simulink library "VIS_LIB"  (Simulink 8.6)
settings: Solver=ode45  StartTime=0.0  StopTime=10.0  RelTol=1e-3
undefined symbols (not defined in the file): AC, SIXOSEM_F_WD_AC_MASTER
libraries: cdsFilt x376, cdsEpicsOut x253, cdsEpicsIn x179, cdsTP x123, VIS_LIB x95, cdsMuxMatrix x91, cdsEpicsStringIn x75, cdsFiltCtrl x72, cdsFunctionCall x70, cdsRms x59, KAGRA_UTIL x25, STATE_BIO_MASTER x5
(part 3 of 38)

== system VIS_LIB/DIAG_OL ==
  TILT_SEG1_In : Inport
  TILT_SEG2_In : Inport  Port=2
  TILT_SEG3_In : Inport  Port=3
  TILT_SEG4_In : Inport  Port=4
  LEN_SEG1_In : Inport  Port=5
  LEN_SEG2_In : Inport  Port=6
  LEN_SEG3_In : Inport  Port=7
  LEN_SEG4_In : Inport  Port=8
  DECPL : cdsMuxMatrix/Subsystem  Tag=cdsMuxMatrix  Description=Any size matrix. Inputs and outputs must be connected using Mux and Demux parts.
      settings: AttributesFormatString=%<Tag>
  Demux2 : Demux  Outputs=6
  Demux4 : Demux  Outputs=6
  LEN : cdsFilt/Subsystem  Tag=cdsFilt  Description=|
      | Purpose:                                                                                                                                                                                                                                  
      | Standard CDS IIR filter module.                                                                                                                                                                                                           
      |                                                                                                                                                                                                                                           
      | Operation:                                                                                                                                                                                                                                
      | Consists of 10 second order section IIR filters, plus a ramped gain stage. In FE code, also provides pre-defined test points and excitation channel inputs. The filter coefficients are defined in the LIGO system using the 'foton' tool.
      |                                                                                                                                                                                                                                           
      | Usage:                                                                                                                                                                                                                                    
      | Name the part with the desired filter module name.
      settings: AttributesFormatString=%<Tag>
  Mux2 : Mux
  Mux4 : Mux  Inputs=6
  OPLEV_LEN : QPD/QPD_WITH_WHITEN_CTRL
  OPLEV_TILT : QPD/QPD_WITH_WHITEN_CTRL
  PIT : cdsFilt/Subsystem  Tag=cdsFilt  Description=|
      | Purpose:                                                                                                                                                                                                                                  
      | Standard CDS IIR filter module.                                                                                                                                                                                                           
      |                                                                                                                                                                                                                                           
      | Operation:                                                                                                                                                                                                                                
      | Consists of 10 second order section IIR filters, plus a ramped gain stage. In FE code, also provides pre-defined test points and excitation channel inputs. The filter coefficients are defined in the LIGO system using the 'foton' tool.
      |                                                                                                                                                                                                                                           
      | Usage:                                                                                                                                                                                                                                    
      | Name the part with the desired filter module name.
      settings: AttributesFormatString=%<Tag>
  ROL : cdsFilt/Subsystem  Tag=cdsFilt  Description=|
      | Purpose:                                                                                                                                                                                                                                  
      | Standard CDS IIR filter module.                                                                                                                                                                                                           
      |                                                                                                                                                                                                                                           
      | Operation:                                                                                                                                                                                                                                
      | Consists of 10 second order section IIR filters, plus a ramped gain stage. In FE code, also provides pre-defined test points and excitation channel inputs. The filter coefficients are defined in the LIGO system using the 'foton' tool.
      |                                                                                                                                                                                                                                           
      | Usage:                                                                                                                                                                                                                                    
      | Name the part with the desired filter module name.
      settings: AttributesFormatString=%<Tag>
  SEN2EUL : cdsMuxMatrix/Subsystem  Tag=cdsMuxMatrix  Description=Any size matrix. Inputs and outputs must be connected using Mux and Demux parts.
      settings: AttributesFormatString=%<Tag>
  TRA : cdsFilt/Subsystem  Tag=cdsFilt  Description=|
      | Purpose:                                                                                                                                                                                                                                  
      | Standard CDS IIR filter module.                                                                                                                                                                                                           
      |                                                                                                                                                                                                                                           
      | Operation:                                                                                                                                                                                                                                
      | Consists of 10 second order section IIR filters, plus a ramped gain stage. In FE code, also provides pre-defined test points and excitation channel inputs. The filter coefficients are defined in the LIGO system using the 'foton' tool.
      |                                                                                                                                                                                                                                           
      | Usage:                                                                                                                                                                                                                                    
      | Name the part with the desired filter module name.
      settings: AttributesFormatString=%<Tag>
  Terminator{1..2,5..8,50..52,54} (10 alike) : Terminator
  VER : cdsFilt/Subsystem  Tag=cdsFilt  Description=|
      | Purpose:                                                                                                                                                                                                                                  
      | Standard CDS IIR filter module.                                                                                                                                                                                                           
      |                                                                                                                                                                                                                                           
      | Operation:                                                                                                                                                                                                                                
      | Consists of 10 second order section IIR filters, plus a ramped gain stage. In FE code, also provides pre-defined test points and excitation channel inputs. The filter coefficients are defined in the LIGO system using the 'foton' tool.
      |                                                                                                                                                                                                                                           
      | Usage:                                                                                                                                                                                                                                    
      | Name the part with the desired filter module name.
      settings: AttributesFormatString=%<Tag>
  YAW : cdsFilt/Subsystem  Tag=cdsFilt  Description=|
      | Purpose:                                                                                                                                                                                                                                  
      | Standard CDS IIR filter module.                                                                                                                                                                                                           
      |                                                                                                                                                                                                                                           
      | Operation:                                                                                                                                                                                                                                
      | Consists of 10 second order section IIR filters, plus a ramped gain stage. In FE code, also provides pre-defined test points and excitation channel inputs. The filter coefficients are defined in the LIGO system using the 'foton' tool.
      |                                                                                                                                                                                                                                           
      | Usage:                                                                                                                                                                                                                                    
      | Name the part with the desired filter module name.
      settings: AttributesFormatString=%<Tag>
  len : Outport
  tra : Outport  Port=2
  ver : Outport  Port=3
  rol : Outport  Port=4
  pit : Outport  Port=5
  yaw : Outport  Port=6
  wires:
  ROL/1 -> rol/1
  PIT/1 -> pit/1
  YAW/1 -> yaw/1
  LEN/1 -> len/1
  TRA/1 -> tra/1
  VER/1 -> ver/1
  Demux2/1 -> LEN/1
  Demux2/2 -> TRA/1
  Demux2/3 -> VER/1
  Demux2/4 -> ROL/1
  Demux2/5 -> PIT/1
  Demux2/6 -> YAW/1
  [LEN_H] -> Mux2/4
  OPLEV_TILT/5 -> Terminator50/1
  OPLEV_TILT/7 -> Terminator52/1
  OPLEV_TILT/6 -> Terminator51/1
  OPLEV_TILT/4 -> Terminator54/1
  OPLEV_TILT/3 -> Terminator1/1
  OPLEV_TILT/1 -> [TILT_V]
  OPLEV_TILT/2 -> [TILT_H]
  TILT_SEG4_In/1 -> OPLEV_TILT/4
  TILT_SEG3_In/1 -> OPLEV_TILT/3
  TILT_SEG2_In/1 -> OPLEV_TILT/2
  TILT_SEG1_In/1 -> OPLEV_TILT/1
  LEN_SEG3_In/1 -> OPLEV_LEN/3
  LEN_SEG2_In/1 -> OPLEV_LEN/2
  LEN_SEG1_In/1 -> OPLEV_LEN/1
  [LEN_V] -> Mux2/3
  OPLEV_LEN/3 -> Terminator2/1
  OPLEV_LEN/1 -> [LEN_V]
  OPLEV_LEN/2 -> [LEN_H]
  LEN_SEG4_In/1 -> OPLEV_LEN/4
  [TILT_V] -> Mux2/1
  OPLEV_LEN/7 -> Terminator7/1
  OPLEV_LEN/6 -> Terminator6/1
  OPLEV_LEN/5 -> Terminator5/1
  OPLEV_LEN/4 -> Terminator8/1
  [TILT_H] -> Mux2/2
  DECPL/1 -> Demux2/1
  Demux4/6 -> Mux4/6
  Mux4/1 -> DECPL/1
  Demux4/4 -> Mux4/4
  Demux4/5 -> Mux4/5
  Demux4/3 -> Mux4/3
  Demux4/2 -> Mux4/2
  Demux4/1 -> Mux4/1
  SEN2EUL/1 -> Demux4/1
  Mux2/1 -> SEN2EUL/1

== system VIS_LIB/DITHER ==
  PIT_In : Inport
  YAW_In : Inport  Port=2
  P : cdsFilt/Subsystem  Tag=cdsFilt  Description=|
      | Purpose:                                                                                                                                                                                                                                  
      | Standard CDS IIR filter module.                                                                                                                                                                                                           
      |                                                                                                                                                                                                                                           
      | Operation:                                                                                                                                                                                                                                
      | Consists of 10 second order section IIR filters, plus a ramped gain stage. In FE code, also provides pre-defined test points and excitation channel inputs. The filter coefficients are defined in the LIGO system using the 'foton' tool.
      |                                                                                                                                                                                                                                           
      | Usage:                                                                                                                                                                                                                                    
      | Name the part with the desired filter module name.
      settings: AttributesFormatString=%<Tag>
  Y : cdsFilt/Subsystem  Tag=cdsFilt  Description=|
      | Purpose:                                                                                                                                                                                                                                  
      | Standard CDS IIR filter module.                                                                                                                                                                                                           
      |                                                                                                                                                                                                                                           
      | Operation:                                                                                                                                                                                                                                
      | Consists of 10 second order section IIR filters, plus a ramped gain stage. In FE code, also provides pre-defined test points and excitation channel inputs. The filter coefficients are defined in the LIGO system using the 'foton' tool.
      |                                                                                                                                                                                                                                           
      | Usage:                                                                                                                                                                                                                                    
      | Name the part with the desired filter module name.
      settings: AttributesFormatString=%<Tag>
  PIT_Out : Outport
  YAW_Out : Outport  Port=2
  wires:
  P/1 -> PIT_Out/1
  YAW_In/1 -> Y/1
  Y/1 -> YAW_Out/1
  PIT_In/1 -> P/1

== system VIS_LIB/DRIVEALIGN ==
  note: This could/should be replaced by
      | the CDS_PART cdsFiltMuxMatrix,
      | but I'm not sure how that works
      | in MEDM land just yet
      | -- JSK Feb 2011
  LONG_In : Inport
  PITCH_In : Inport  Port=2
  YAW_In : Inport  Port=3
  L2L : cdsFilt/Subsystem  Tag=cdsFilt  Description=|
      | Purpose:                                                                                                                                                                                                                                  
      | Standard CDS IIR filter module.                                                                                                                                                                                                           
      |                                                                                                                                                                                                                                           
      | Operation:                                                                                                                                                                                                                                
      | Consists of 10 second order section IIR filters, plus a ramped gain stage. In FE code, also provides pre-defined test points and excitation channel inputs. The filter coefficients are defined in the LIGO system using the 'foton' tool.
      |                                                                                                                                                                                                                                           
      | Usage:                                                                                                                                                                                                                                    
      | Name the part with the desired filter module name.
      settings: AttributesFormatString=%<Tag>
  L2P : cdsFilt/Subsystem  Tag=cdsFilt  Description=|
      | Purpose:                                                                                                                                                                                                                                  
      | Standard CDS IIR filter module.                                                                                                                                                                                                           
      |                                                                                                                                                                                                                                           
      | Operation:                                                                                                                                                                                                                                
      | Consists of 10 second order section IIR filters, plus a ramped gain stage. In FE code, also provides pre-defined test points and excitation channel inputs. The filter coefficients are defined in the LIGO system using the 'foton' tool.
      |                                                                                                                                                                                                                                           
      | Usage:                                                                                                                                                                                                                                    
      | Name the part with the desired filter module name.
      settings: AttributesFormatString=%<Tag>
  L2Y : cdsFilt/Subsystem  Tag=cdsFilt  Description=|
      | Purpose:                                                                                                                                                                                                                                  
      | Standard CDS IIR filter module.                                                                                                                                                                                                           
      |                                                                                                                                                                                                                                           
      | Operation:                                                                                                                                                                                                                                
      | Consists of 10 second order section IIR filters, plus a ramped gain stage. In FE code, also provides pre-defined test points and excitation channel inputs. The filter coefficients are defined in the LIGO system using the 'foton' tool.
      |                                                                                                                                                                                                                                           
      | Usage:                                                                                                                                                                                                                                    
      | Name the part with the desired filter module name.
      settings: AttributesFormatString=%<Tag>
  L_IN : cdsTP/Subsystem  Tag=Test Point
      settings: AttributesFormatString=%<Tag>
  L_INMON : cdsEpicsOut/Subsystem  Tag=cdsEpicsOutput  Description=|
      | Purpose:                                          
      | Output a FE signal to an EPICS channel.           
      |                                                   
      | Operation:                                        
      | Takes input value and passes it to EPICS record.  
      |                                                   
      | Usage:                                            
      | Name the part with the desired EPICS rrecord name.
      settings: AttributesFormatString=%<Tag>
  L_OUT : cdsTP/Subsystem  Tag=Test Point
      settings: AttributesFormatString=%<Tag>
  L_OUTMON : cdsEpicsOut/Subsystem  Tag=cdsEpicsOutput  Description=|
      | Purpose:                                          
      | Output a FE signal to an EPICS channel.           
      |                                                   
      | Operation:                                        
      | Takes input value and passes it to EPICS record.  
      |                                                   
      | Usage:                                            
      | Name the part with the desired EPICS rrecord name.
      settings: AttributesFormatString=%<Tag>
  P2L : cdsFilt/Subsystem  Tag=cdsFilt  Description=|
      | Purpose:                                                                                                                                                                                                                                  
      | Standard CDS IIR filter module.                                                                                                                                                                                                           
      |                                                                                                                                                                                                                                           
      | Operation:                                                                                                                                                                                                                                
      | Consists of 10 second order section IIR filters, plus a ramped gain stage. In FE code, also provides pre-defined test points and excitation channel inputs. The filter coefficients are defined in the LIGO system using the 'foton' tool.
      |                                                                                                                                                                                                                                           
      | Usage:                                                                                                                                                                                                                                    
      | Name the part with the desired filter module name.
      settings: AttributesFormatString=%<Tag>
  P2P : cdsFilt/Subsystem  Tag=cdsFilt  Description=|
      | Purpose:                                                                                                                                                                                                                                  
      | Standard CDS IIR filter module.                                                                                                                                                                                                           
      |                                                                                                                                                                                                                                           
      | Operation:                                                                                                                                                                                                                                
      | Consists of 10 second order section IIR filters, plus a ramped gain stage. In FE code, also provides pre-defined test points and excitation channel inputs. The filter coefficients are defined in the LIGO system using the 'foton' tool.
      |                                                                                                                                                                                                                                           
      | Usage:                                                                                                                                                                                                                                    
      | Name the part with the desired filter module name.
      settings: AttributesFormatString=%<Tag>
  P2Y : cdsFilt/Subsystem  Tag=cdsFilt  Description=|
      | Purpose:                                                                                                                                                                                                                                  
      | Standard CDS IIR filter module.                                                                                                                                                                                                           
      |                                                                                                                                                                                                                                           
      | Operation:                                                                                                                                                                                                                                
      | Consists of 10 second order section IIR filters, plus a ramped gain stage. In FE code, also provides pre-defined test points and excitation channel inputs. The filter coefficients are defined in the LIGO system using the 'foton' tool.
      |                                                                                                                                                                                                                                           
      | Usage:                                                                                                                                                                                                                                    
      | Name the part with the desired filter module name.
      settings: AttributesFormatString=%<Tag>
  P_IN : cdsTP/Subsystem  Tag=Test Point
      settings: AttributesFormatString=%<Tag>
  P_INMON : cdsEpicsOut/Subsystem  Tag=cdsEpicsOutput  Description=|
      | Purpose:                                          
      | Output a FE signal to an EPICS channel.           
      |                                                   
      | Operation:                                        
      | Takes input value and passes it to EPICS record.  
      |                                                   
      | Usage:                                            
      | Name the part with the desired EPICS rrecord name.
      settings: AttributesFormatString=%<Tag>
  P_OUT : cdsTP/Subsystem  Tag=Test Point
      settings: AttributesFormatString=%<Tag>
  P_OUTMON : cdsEpicsOut/Subsystem  Tag=cdsEpicsOutput  Description=|
      | Purpose:                                          
      | Output a FE signal to an EPICS channel.           
      |                                                   
      | Operation:                                        
      | Takes input value and passes it to EPICS record.  
      |                                                   
      | Usage:                                            
      | Name the part with the desired EPICS rrecord name.
      settings: AttributesFormatString=%<Tag>
  Sum : Sum  Inputs=+++
  Sum1 : Sum  Inputs=+++
  Sum2 : Sum  Inputs=+++
  Y2L : cdsFilt/Subsystem  Tag=cdsFilt  Description=|
      | Purpose:                                                                                                                                                                                                                                  
      | Standard CDS IIR filter module.                                                                                                                                                                                                           
      |                                                                                                                                                                                                                                           
      | Operation:                                                                                                                                                                                                                                
      | Consists of 10 second order section IIR filters, plus a ramped gain stage. In FE code, also provides pre-defined test points and excitation channel inputs. The filter coefficients are defined in the LIGO system using the 'foton' tool.
      |                                                                                                                                                                                                                                           
      | Usage:                                                                                                                                                                                                                                    
      | Name the part with the desired filter module name.
      settings: AttributesFormatString=%<Tag>
  Y2P : cdsFilt/Subsystem  Tag=cdsFilt  Description=|
      | Purpose:                                                                                                                                                                                                                                  
      | Standard CDS IIR filter module.                                                                                                                                                                                                           
      |                                                                                                                                                                                                                                           
      | Operation:                                                                                                                                                                                                                                
      | Consists of 10 second order section IIR filters, plus a ramped gain stage. In FE code, also provides pre-defined test points and excitation channel inputs. The filter coefficients are defined in the LIGO system using the 'foton' tool.
      |                                                                                                                                                                                                                                           
      | Usage:                                                                                                                                                                                                                                    
      | Name the part with the desired filter module name.
      settings: AttributesFormatString=%<Tag>
  Y2Y : cdsFilt/Subsystem  Tag=cdsFilt  Description=|
      | Purpose:                                                                                                                                                                                                                                  
      | Standard CDS IIR filter module.                                                                                                                                                                                                           
      |                                                                                                                                                                                                                                           
      | Operation:                                                                                                                                                                                                                                
      | Consists of 10 second order section IIR filters, plus a ramped gain stage. In FE code, also provides pre-defined test points and excitation channel inputs. The filter coefficients are defined in the LIGO system using the 'foton' tool.
      |                                                                                                                                                                                                                                           
      | Usage:                                                                                                                                                                                                                                    
      | Name the part with the desired filter module name.
      settings: AttributesFormatString=%<Tag>
  Y_IN : cdsTP/Subsystem  Tag=Test Point
      settings: AttributesFormatString=%<Tag>
  Y_INMON : cdsEpicsOut/Subsystem  Tag=cdsEpicsOutput  Description=|
      | Purpose:                                          
      | Output a FE signal to an EPICS channel.           
      |                                                   
      | Operation:                                        
      | Takes input value and passes it to EPICS record.  
      |                                                   
      | Usage:                                            
      | Name the part with the desired EPICS rrecord name.
      settings: AttributesFormatString=%<Tag>
  Y_OUT : cdsTP/Subsystem  Tag=Test Point
      settings: AttributesFormatString=%<Tag>
  Y_OUTMON : cdsEpicsOut/Subsystem  Tag=cdsEpicsOutput  Description=|
      | Purpose:                                          
      | Output a FE signal to an EPICS channel.           
      |                                                   
      | Operation:                                        
      | Takes input value and passes it to EPICS record.  
      |                                                   
      | Usage:                                            
      | Name the part with the desired EPICS rrecord name.
      settings: AttributesFormatString=%<Tag>
  LONG_Out : Outport
  PITCH_Out : Outport  Port=2
  YAW_Out : Outport  Port=3
  wires:
  Y_OUTMON/1 -> YAW_Out/1
  P_OUTMON/1 -> PITCH_Out/1
  L_OUTMON/1 -> LONG_Out/1
  Y_INMON/1 -> Y_IN/1, Y2L/1, Y2Y/1, Y2P/1
  P_INMON/1 -> P_IN/1, P2L/1, P2Y/1, P2P/1
  L_INMON/1 -> L_IN/1, L2Y/1, L2P/1, L2L/1
  L2L/1 -> Sum/1
  P2L/1 -> Sum/2
  Y2L/1 -> Sum/3
  Y2P/1 -> Sum1/3
  P2P/1 -> Sum1/2
  L2P/1 -> Sum1/1
  Y2Y/1 -> Sum2/3
  P2Y/1 -> Sum2/2
  L2Y/1 -> Sum2/1
  Sum/1 -> L_OUT/1, L_OUTMON/1
  Sum1/1 -> P_OUT/1, P_OUTMON/1
  Sum2/1 -> Y_OUT/1, Y_OUTMON/1
  LONG_In/1 -> L_INMON/1
  PITCH_In/1 -> P_INMON/1
  YAW_In/1 -> Y_INMON/1

== system VIS_LIB/EULOUT ==
  LONG_In : Inport
  TRANS_In : Inport  Port=2
  VERT_In : Inport  Port=3
  ROLL_In : Inport  Port=4
  PITCH_In : Inport  Port=5
  YAW_In : Inport  Port=6
  L : cdsTP/Subsystem  Tag=Test Point
      settings: AttributesFormatString=%<Tag>
  L_MON : cdsEpicsOut/Subsystem  Tag=cdsEpicsOutput  Description=|
      | Purpose:                                          
      | Output a FE signal to an EPICS channel.           
      |                                                   
      | Operation:                                        
      | Takes input value and passes it to EPICS record.  
      |                                                   
      | Usage:                                            
      | Name the part with the desired EPICS rrecord name.
      settings: AttributesFormatString=%<Tag>
  P : cdsTP/Subsystem  Tag=Test Point
      settings: AttributesFormatString=%<Tag>
  P_MON : cdsEpicsOut/Subsystem  Tag=cdsEpicsOutput  Description=|
      | Purpose:                                          
      | Output a FE signal to an EPICS channel.           
      |                                                   
      | Operation:                                        
      | Takes input value and passes it to EPICS record.  
      |                                                   
      | Usage:                                            
      | Name the part with the desired EPICS rrecord name.
      settings: AttributesFormatString=%<Tag>
  R : cdsTP/Subsystem  Tag=Test Point
      settings: AttributesFormatString=%<Tag>
  R_MON : cdsEpicsOut/Subsystem  Tag=cdsEpicsOutput  Description=|
      | Purpose:                                          
      | Output a FE signal to an EPICS channel.           
      |                                                   
      | Operation:                                        
      | Takes input value and passes it to EPICS record.  
      |                                                   
      | Usage:                                            
      | Name the part with the desired EPICS rrecord name.
      settings: AttributesFormatString=%<Tag>
  T : cdsTP/Subsystem  Tag=Test Point
      settings: AttributesFormatString=%<Tag>
  T_MON : cdsEpicsOut/Subsystem  Tag=cdsEpicsOutput  Description=|
      | Purpose:                                          
      | Output a FE signal to an EPICS channel.           
      |                                                   
      | Operation:                                        
      | Takes input value and passes it to EPICS record.  
      |                                                   
      | Usage:                                            
      | Name the part with the desired EPICS rrecord name.
      settings: AttributesFormatString=%<Tag>
  V : cdsTP/Subsystem  Tag=Test Point
      settings: AttributesFormatString=%<Tag>
  V_MON : cdsEpicsOut/Subsystem  Tag=cdsEpicsOutput  Description=|
      | Purpose:                                          
      | Output a FE signal to an EPICS channel.           
      |                                                   
      | Operation:                                        
      | Takes input value and passes it to EPICS record.  
      |                                                   
      | Usage:                                            
      | Name the part with the desired EPICS rrecord name.
      settings: AttributesFormatString=%<Tag>
  Y : cdsTP/Subsystem  Tag=Test Point
      settings: AttributesFormatString=%<Tag>
  Y_MON : cdsEpicsOut/Subsystem  Tag=cdsEpicsOutput  Description=|
      | Purpose:                                          
      | Output a FE signal to an EPICS channel.           
      |                                                   
      | Operation:                                        
      | Takes input value and passes it to EPICS record.  
      |                                                   
      | Usage:                                            
      | Name the part with the desired EPICS rrecord name.
      settings: AttributesFormatString=%<Tag>
  wires:
  T_MON/1 -> T/1
  TRANS_In/1 -> T_MON/1
  Y_MON/1 -> Y/1
  YAW_In/1 -> Y_MON/1
  L_MON/1 -> L/1
  LONG_In/1 -> L_MON/1
  R_MON/1 -> R/1
  ROLL_In/1 -> R_MON/1
  V_MON/1 -> V/1
  VERT_In/1 -> V_MON/1
  P_MON/1 -> P/1
  PITCH_In/1 -> P_MON/1

== system VIS_LIB/ISCINF ==
  LONG_In : Inport
  PITCH_In : Inport  Port=2
  YAW_In : Inport  Port=3
  L : cdsFilt/Subsystem  Tag=cdsFilt  Description=|
      | Purpose:                                                                                                                                                                                                                                  
      | Standard CDS IIR filter module.                                                                                                                                                                                                           
      |                                                                                                                                                                                                                                           
      | Operation:                                                                                                                                                                                                                                
      | Consists of 10 second order section IIR filters, plus a ramped gain stage. In FE code, also provides pre-defined test points and excitation channel inputs. The filter coefficients are defined in the LIGO system using the 'foton' tool.
      |                                                                                                                                                                                                                                           
      | Usage:                                                                                                                                                                                                                                    
      | Name the part with the desired filter module name.
      settings: AttributesFormatString=%<Tag>
  P : cdsFilt/Subsystem  Tag=cdsFilt  Description=|
      | Purpose:                                                                                                                                                                                                                                  
      | Standard CDS IIR filter module.                                                                                                                                                                                                           
      |                                                                                                                                                                                                                                           
      | Operation:                                                                                                                                                                                                                                
      | Consists of 10 second order section IIR filters, plus a ramped gain stage. In FE code, also provides pre-defined test points and excitation channel inputs. The filter coefficients are defined in the LIGO system using the 'foton' tool.
      |                                                                                                                                                                                                                                           
      | Usage:                                                                                                                                                                                                                                    
      | Name the part with the desired filter module name.
      settings: AttributesFormatString=%<Tag>
  Y : cdsFilt/Subsystem  Tag=cdsFilt  Description=|
      | Purpose:                                                                                                                                                                                                                                  
      | Standard CDS IIR filter module.                                                                                                                                                                                                           
      |                                                                                                                                                                                                                                           
      | Operation:                                                                                                                                                                                                                                
      | Consists of 10 second order section IIR filters, plus a ramped gain stage. In FE code, also provides pre-defined test points and excitation channel inputs. The filter coefficients are defined in the LIGO system using the 'foton' tool.
      |                                                                                                                                                                                                                                           
      | Usage:                                                                                                                                                                                                                                    
      | Name the part with the desired filter module name.
      settings: AttributesFormatString=%<Tag>
  LONG_Out : Outport
  PITCH_Out : Outport  Port=2
  YAW_Out : Outport  Port=3
  wires:
  L/1 -> LONG_Out/1
  Y/1 -> YAW_Out/1
  P/1 -> PITCH_Out/1
  LONG_In/1 -> L/1
  YAW_In/1 -> Y/1
  PITCH_In/1 -> P/1
